simulink model "quadcopterModel"  (R2018b)
settings: Solver=ode1  StartTime=0.0  StopTime=param.tfinal  FixedStep=param.dt  RelTol=1e-3
values from neighbouring files (symbols this model uses):
  acc_acom = [1 om_com]    [quadSimRunMain.m]
  acc_bcom = [0 om_com]    [quadSimRunMain.m]
  agyro = 1    [quadSimRunMain.m]
  bgyro = 1    [quadSimRunMain.m]
  gainAcc = 1    [quadSimRunMain.m]
  gainGyro = 1    [quadSimRunMain.m]
  gainPsi = 1    [quadSimRunMain.m]
  gainWind = 1    [quadSimRunMain.m]
  gyro_acom = [1 om_com]    [quadSimRunMain.m]
  gyro_bcom = [1 0]    [quadSimRunMain.m]
  Kdphi = 0.0478*1    (= 0.0478)    [quadSimRunMain.m]
  Kdpsi = 0.067644*1    (= 0.067644)    [quadSimRunMain.m]
  Kdtheta = 0.0478*1    (= 0.0478)    [quadSimRunMain.m]
  Kdx = 15    [quadSimRunMain.m]
  Kdy = 15    [quadSimRunMain.m]
  Kdz = 5.5    [quadSimRunMain.m]
  Kiphi = 0.0098*0    (= 0)    [quadSimRunMain.m]
  Kipsi = 0.045028*.0    (= 0)    [quadSimRunMain.m]
  Kitheta = 0.0098*0    (= 0)    [quadSimRunMain.m]
  Kix = 1    [quadSimRunMain.m]
  Kiy = 1    [quadSimRunMain.m]
  Kiz = 1.5    [quadSimRunMain.m]
  Kpphi = 0.0439*1    (= 0.0439)    [quadSimRunMain.m]
  Kppsi = 0.11038*1    (= 0.11038)    [quadSimRunMain.m]
  Kptheta = 0.0439*1    (= 0.0439)    [quadSimRunMain.m]
  Kpx = 5    [quadSimRunMain.m]
  Kpy = 5    [quadSimRunMain.m]
  Kpz = 3.5    [quadSimRunMain.m]
  Nphi = 1/Tfphi    (= 162.638649449)    [quadSimRunMain.m]
  Npsi = 1/Tfpsi    (= 159.182438993)    [quadSimRunMain.m]
  Ntheta = 1/Tftheta    (= 162.638649449)    [quadSimRunMain.m]
  Nx = 1/0.002099    (= 476.417341591)    [quadSimRunMain.m]
  Ny = 1/0.002099    (= 476.417341591)    [quadSimRunMain.m]
  Nz = 1/0.002099    (= 476.417341591)    [quadSimRunMain.m]
  param = quadparam    [quadDyn.m]    (also in quadDynSimple.m; quadSimRunMain.m; quadcomputeFandT.m; quadcomputeMotorSpeed.m)
  pathSelect = 1    [quadSimRunMain.m]
  windConstant = 1    [quadSimRunMain.m]
  windVarying = 1    [quadSimRunMain.m]
undefined symbols (not defined in the file or in its folder): aHu, aHv, aHw, bHu, bHv, bHw, DiscIntNeverNeededParam
libraries: simulink x7, sharedutil x4
(part 2 of 2)

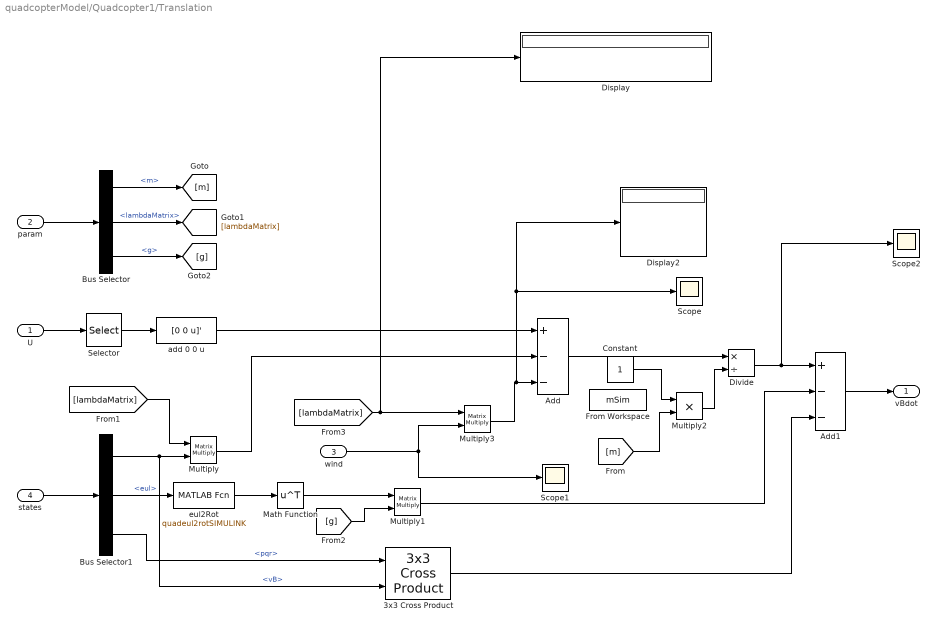
== system quadcopterModel/Quadcopter1/Translation ==
  U : Inport
  param : Inport  Port=2
  wind : Inport  Port=3
  states : Inport  Port=4
  3x3 Cross Product : sharedutil/3x3 Cross Product  aMode=aMode
      settings: SourceProductBaseCode=AE
  Add : Sum  Inputs=+--
  Add1 : Sum  Inputs=+--
  Bus Selector : BusSelector  OutputSignals=m,lambdaMatrix,g
  Bus Selector1 : BusSelector  OutputSignals=vB,eul,pqr
  Constant : Constant
  Display : Display
  Display2 : Display
  Divide : Product  Inputs=*/
  From Workspace : FromWorkspace  VariableName=mSim  SampleTime=0
  Math Function : Math  Operator=transpose  SaturateOnIntegerOverflow=on
  Multiply : Product  Multiplication=Matrix(*)
  Multiply1 : Product  Multiplication=Matrix(*)
  Multiply2 : Product
  Multiply3 : Product  Multiplication=Matrix(*)
  Scope : Scope
  Scope1 : Scope
  Scope2 : Scope
  Selector : Selector  InputPortWidth=4  IndexOptions=Index vector (dialog)  Indices=1  OutputSizes=1
  add 0 0 u : MATLABFcn  MATLABFcn=[0 0 u]'
  eul2Rot : MATLABFcn  MATLABFcn=quadeul2rotSIMULINK  OutputDimensions=[3 3]  OutputSignalType=real  Output1D=off
  vBdot : Outport
  wires:
  [m] -> Multiply2/2
  Multiply2/1 -> Divide/2
  wind/1 -> Scope1/1, Multiply3/2
  eul2Rot/1 -> Math Function/1
  3x3 Cross Product/1 -> Add1/3
  Bus Selector1/3 -> 3x3 Cross Product/1  "<pqr>"
  Multiply3/1 -> Add/3, Scope/1, Display2/1
  [lambdaMatrix] -> Multiply3/1, Display/1
  Math Function/1 -> Multiply1/1
  Add1/1 -> vBdot/1
  Multiply1/1 -> Add1/2
  Divide/1 -> Add1/1, Scope2/1
  [g] -> Multiply1/2
  Bus Selector1/2 -> eul2Rot/1  "<eul>"
  Multiply/1 -> Add/2
  [lambdaMatrix] -> Multiply/1
  Bus Selector1/1 -> Multiply/2, 3x3 Cross Product/2  "<vB>"
  states/1 -> Bus Selector1/1
  Add/1 -> Divide/1
  add 0 0 u/1 -> Add/1
  Bus Selector/3 -> [g]  "<g>"
  Bus Selector/2 -> [lambdaMatrix]  "<lambdaMatrix>"
  Bus Selector/1 -> [m]  "<m>"
  param/1 -> Bus Selector/1
  Selector/1 -> add 0 0 u/1
  U/1 -> Selector/1
  Constant/1 -> Multiply2/1

== system quadcopterModel/Quadcopter1/addNoiseToIMU ==
  a_noNoise : Inport
  gyr_noNoise : Inport  Port=2
  Add : Sum
  Add1 : Sum
  Demux : Demux  Outputs=3
  From Workspace : FromWorkspace  VariableName=eacc  SampleTime=0
  From Workspace1 : FromWorkspace  VariableName=egyro  SampleTime=0
  Gain : Gain  Gain=0
  Gain1 : Gain  Gain=0
  Mux : Mux  Inputs=3
  Transfer Fcn : TransferFcn  Numerator=bgyro  Denominator=agyro
  Transfer Fcn1 : TransferFcn  Numerator=bgyro  Denominator=agyro
  Transfer Fcn2 : TransferFcn  Numerator=bgyro  Denominator=agyro
  acc : Outport
  gyro : Outport  Port=2
  gyro0 : Outport  Port=3
  wires:
  Add1/1 -> gyro/1  "gyro"
  From Workspace/1 -> Gain/1
  a_noNoise/1 -> Add/2
  gyr_noNoise/1 -> gyro0/1, Add1/2
  Add/1 -> acc/1  "acc"
  From Workspace1/1 -> Demux/1
  Demux/1 -> Transfer Fcn/1
  Demux/2 -> Transfer Fcn1/1
  Demux/3 -> Transfer Fcn2/1
  Transfer Fcn/1 -> Mux/1
  Transfer Fcn1/1 -> Mux/2
  Transfer Fcn2/1 -> Mux/3
  Mux/1 -> Gain1/1
  Gain/1 -> Add/1
  Gain1/1 -> Add1/1

== matlab function quadcopterModel/Path Generation/Compute Psi from trajectory/MATLAB Function ==
  data: xydot input; psi output; psiOld input; psiPure output; epsi output
function [psi, psiPure,epsi] = fcn(xydot, psiOld)


xdot = xydot(1);ydot = xydot(2);
psi = atan2(ydot,xdot);
psiPure = psi;



if psi-psiOld>6 && psi-psiOld<10
    psi = psi-2*pi;
end
if psi-psiOld>10
    psi = psi - 4*pi;
end
if psi-psiOld<-6 && psi-psiOld>-10
    psi = psi+2*pi;
end
if psi-psiOld<-10
    psi = psi+4*pi;
end
% if psi>3 && psi-psiOld>3
%     psi = psi-2*pi;
% end
% if psi<-3 && psi-psiOld<-3
%     psi = psi + 2*pi;
% end
epsi = psi-psiOld;

== matlab function quadcopterModel/QuadSimpifiedModel/quadDynComplex ==
  data: velocities input; eul input; U input; V_W input; pddot output; eulddot output; pddot0w output; ameas output
function [pddot, eulddot, pddot0w, ameas] = quadDynComplex(velocities,eul,U,V_W)
%quadDynSimple Simplified translation and rotation of quadcopter
%   euler: the Euler angles of quadcopter
%   U: The control signal around trim condition: U_z tau_phi tau_theta
%   tau_psi
%   V_W: wind velocity: u_w v_w w_w

param.m = 0.5;
param.g = [0 0 9.81]';
param.cd = 0.32;
param.cf = 1e-4;
param.L = 0.5;
param.ct = 1e-5;
param.Jx = 0.002;
param.Jy = 0.002;
param.Jz = 0.003;
param.lambda1 = 0.36;
param.lambda2 = 0.6;
param.alpha1 = 0.002;
param.alpha2 = 0.005;

param.alphaphi = 0.002;

pdot = velocities(1:3);
eulerdot = velocities(4:6);
u_w = V_W(1);v_w = V_W(2);w_w = V_W(3);
Seuldot = [0 -eulerdot(3) eulerdot(2);...
    eulerdot(3) 0 -eulerdot(1);...
    -eulerdot(2) eulerdot(1) 0];

% Compute the translational and rotational acceleartions with wind effect
ameas= 1/param.m*([0 0 U(1)]' - [param.lambda1*(pdot(1)+u_w);...
    param.lambda1*(pdot(2)+v_w); param.lambda2*(pdot(3)+w_w)]);

pddot = ameas + param.g(3)*[eul(2); -eul(1); -1] - 0*Seuldot*pdot;
ameas = ameas; % Have a form of a - g

JJ = diag([param.Jx, param.Jy, param.Jz]);
eulddot = [U(2)/param.Jx ; U(3)/param.Jy - 0*param.alphaphi*u_w/param.Jy; U(4)/param.Jz] -...
    [param.alpha1*eulerdot(1)/param.Jx; param.alpha1*eulerdot(2)/param.Jy;...
    param.alpha2*eulerdot(3)/param.Jz] - 0*inv(JJ)*Seuldot*(JJ*eulerdot);

% Compute the translational and rotational acceleartions without wind effect
pddotn = 1/param.m*([0 0 U(1)]' - param.lambda1*[pdot(1)+0; pdot(2)+0;...
    param.lambda2/param.lambda1*(pdot(3)+0)]) + ...
    param.g(3)*[eul(2); -eul(1); -1];
pddot0w = [pddotn;eulddot];
end

== matlab function quadcopterModel/QuadSimpifiedModel/Rotxy2body ==
  data: eul input; Rpsi output
function Rpsi = rotPsi(eul)
phi = eul(1);theta = eul(2);psi = eul(3);
% Rpsi = [cos(psi) -sin(psi) theta;sin(psi) cos(psi) -phi;-theta phi 1];
Rpsi = [cos(psi) -sin(psi) 0;sin(psi) cos(psi) 0;0 0 1];

== matlab function quadcopterModel/Quadcopter/MATLAB Function1 ==
  data: u input; y output
function y = fcn(u)
y = u;
if y(3)<=0
    y(3) = 0;
end

== matlab function quadcopterModel/QuadSimpifiedModel/eul2T ==
  data: eul input; Rpsi output
function Rpsi = eul2T(eul)
phi = eul(1);theta = eul(2);psi = eul(3);
Rpsi = [1 0 theta;0 1 -phi;0 phi 1];
% Rpsi = eye(3);

== matlab function quadcopterModel/Quadcopter1/MATLAB Function1 ==
  data: u input; y output
function y = fcn(u)
y = u;
if y(3)<=0
    y(3) = 0;
end
